simulink model "sampleModel7288_pp_1_1"  (R2018a)
settings: Solver=VariableStepAuto  StartTime=0.0  StopTime=10.0  RelTol=1e-3
undefined symbols (not defined in the file): DiscIntNeverNeededParam, sigbuilder_block
libraries: simulink x497
(part 5 of 10)

== system sampleModel7288_pp_1_1/cfblk302 ==
  cfblk1 : Inport
  Action Port : ActionPort  ActionType=then
  cfblk{4,7,9..10} (4 alike) : Delay
  cfblk3 : Delay  DelayLengthSource=Input port
      settings: InputPortMap=u0,p1
  cfblk5 : simulink/Discrete/Transfer Fcn Lead or Lag  PoleZ=0.95  ZeroZ=0.75  ICPrevOutput=0.0  ICPrevInput=0.0  DoSatur=off
      settings: SourceProductName=Simulink  SourceProductBaseCode=SL
  cfblk6 : simulink/Discrete/Difference  ICPrevInput=0.0  OutMin=[]  OutMax=[]  OutDataTypeStr=double  OutputDataTypeScalingMode=double  OutDataType=fixdt(1, 16)  OutScaling=2^-10  DoSatur=off
  cyemi_{1236..1243} (8 alike) : DataTypeConversion  OutDataTypeStr=double
  cfblk2 : Outport
  cfblk8 : Outport  Port=2
  wires:
  cfblk1/1 -> cfblk8/1
  cfblk7/1 -> cyemi_1236/1, cyemi_1237/1
  cfblk4/1 -> cyemi_1241/1, cyemi_1242/1
  cfblk6/1 -> cfblk2/1
  cyemi_1236/1 -> cfblk10/1
  cyemi_1237/1 -> cfblk3/1
  cyemi_1238/1 -> cfblk3/2
  cfblk9/1 -> cyemi_1238/1
  cyemi_1239/1 -> cfblk4/1
  cfblk10/1 -> cyemi_1239/1
  cyemi_1240/1 -> cfblk5/1
  cfblk3/1 -> cyemi_1240/1
  cyemi_1241/1 -> cfblk6/1
  cyemi_1242/1 -> cfblk7/1
  cyemi_1243/1 -> cfblk9/1
  cfblk5/1 -> cyemi_1243/1

== system sampleModel7288_pp_1_1/cfblk303 ==
  cfblk1 : Inport
  cfblk13 : Inport  Port=2
  cfblk14 : Inport  Port=3
  cfblk15 : Inport  Port=4
  Action Port : ActionPort  ActionType=else
  cfblk10 : Delay
  cfblk11 : DiscreteIntegrator  SampleTime=-1  OutDataTypeStr=double  ICPrevOutput=DiscIntNeverNeededParam  ICPrevScaledInput=DiscIntNeverNeededParam
  cfblk12 : simulink/Discrete/Transfer Fcn Lead or Lag  PoleZ=0.95  ZeroZ=0.75  ICPrevOutput=0.0  ICPrevInput=0.0  DoSatur=off
      settings: SourceProductName=Simulink  SourceProductBaseCode=SL
  cfblk17 : Delay
  cfblk3 : DiscreteFir
  cfblk4 : DiscreteFir
  cfblk5 : DiscreteStateSpace  SampleTime=-1
  cfblk6 : simulink/Discrete/Transfer Fcn Lead or Lag  PoleZ=0.95  ZeroZ=0.75  ICPrevOutput=0.0  ICPrevInput=0.0  DoSatur=off
      settings: SourceProductName=Simulink  SourceProductBaseCode=SL
  cfblk7 : Delay
  cfblk8 : DiscreteFilter
  cfblk9 : simulink/Discrete/Transfer Fcn Real Zero  ZeroZ=0.75  ICPrevInput=0.0  DoSatur=off
      settings: SourceProductName=Simulink  SourceProductBaseCode=SL
  cyemi_{1248..1258} (11 alike) : DataTypeConversion  OutDataTypeStr=double
  cfblk2 : Outport
  cfblk16 : Outport  Port=2
  wires:
  cfblk14/1 -> cfblk16/1
  cfblk3/1 -> cfblk2/1
  cyemi_1248/1 -> cfblk10/1
  cfblk8/1 -> cyemi_1248/1
  cyemi_1249/1 -> cfblk11/1
  cfblk9/1 -> cyemi_1249/1
  cyemi_1250/1 -> cfblk12/1
  cfblk5/1 -> cyemi_1250/1
  cyemi_1251/1 -> cfblk17/1
  cfblk11/1 -> cyemi_1251/1
  cyemi_1252/1 -> cfblk3/1
  cfblk7/1 -> cyemi_1252/1
  cyemi_1253/1 -> cfblk4/1
  cfblk12/1 -> cyemi_1253/1
  cyemi_1254/1 -> cfblk5/1
  cfblk1/1 -> cyemi_1254/1
  cyemi_1255/1 -> cfblk6/1
  cfblk4/1 -> cyemi_1255/1
  cyemi_1256/1 -> cfblk7/1
  cfblk6/1 -> cyemi_1256/1
  cyemi_1257/1 -> cfblk8/1
  cfblk15/1 -> cyemi_1257/1
  cyemi_1258/1 -> cfblk9/1
  cfblk17/1 -> cyemi_1258/1

== system sampleModel7288_pp_1_1/cfblk304 ==
  cfblk1 : Inport
  cfblk8 : Inport  Port=2
  Action Port : ActionPort  ActionType=then
  cfblk3 : simulink/Discrete/Transfer Fcn First Order  PoleZ=0.95  ICPrevOutput=0.0  DoSatur=off
      settings: SourceProductName=Simulink
  cfblk4 : simulink/Continuous/PID Controller (2DOF)  Controller=PID  TimeDomain=Discrete-time  SampleTime=-1  IntegratorMethod=Forward Euler  FilterMethod=Forward Euler  Form=Parallel  UseFilter=on  ControllerParametersSource=internal  P=1  I=1  D=0  N=100  b=1  c=1  InitialConditionSource=internal  InitialConditionForIntegrator=0  InitialConditionForFilter=0  ExternalReset=none  LimitOutput=off  UpperSaturationLimit=inf  LowerSaturationLimit=-inf  LinearizeAsGain=off  AntiWindupMode=none  Kb=1  TrackingMode=off  Kt=1  PParamMin=[]  PParamMax=[]  IParamMin=[]  IParamMax=[]  DParamMin=[]  DParamMax=[]  NParamMin=[]  NParamMax=[]  bParamMin=[]  bParamMax=[]  cParamMin=[]  cParamMax=[]  KbParamMin=[]  KbParamMax=[]  KtParamMin=[]  KtParamMax=[]  POutMin=[]  POutMax=[]  IOutMin=[]  IOutMax=[]  DOutMin=[]  DOutMax=[]  NOutMin=[]  NOutMax=[]  bOutMin=[]  bOutMax=[]  cOutMin=[]  cOutMax=[]  KbOutMin=[]  KbOutMax=[]  KtOutMin=[]  KtOutMax=[]  IntegratorOutMin=[]  IntegratorOutMax=[]  FilterOutMin=[]  FilterOutMax=[]  SumOutMin=[]  SumOutMax=[]  Sum1OutMin=[]  Sum1OutMax=[]  Sum2OutMin=[]  Sum2OutMax=[]  Sum3OutMin=[]  Sum3OutMax=[]  SumI1OutMin=[]  SumI1OutMax=[]  SumI2OutMin=[]  SumI2OutMax=[]  SumI3OutMin=[]  SumI3OutMax=[]  SumDOutMin=[]  SumDOutMax=[]  SaturationOutMin=[]  SaturationOutMax=[]  IntegratorContinuousStateAttributes=''  IntegratorStateMustResolveToSignalObject=off  IntegratorRTWStateStorageClass=Auto  FilterContinuousStateAttributes=''  FilterStateMustResolveToSignalObject=off  FilterRTWStateStorageClass=Auto  DifferentiatorICPrevScaledInput=0  DifferentiatorOutMin=[]  DifferentiatorOutMax=[]  FilterDiffOutCoefMin=[]  FilterDiffOutCoefMax=[]  SumDenOutMin=[]  SumDenOutMax=[]  SumNumOutMin=[]  SumNumOutMax=[]  ReciprocalOutMin=[]  ReciprocalOutMax=[]  DivideOutMin=[]  DivideOutMax=[]  TunerSelectOption=Transfer Function Based (PID Tuner App)
  cfblk5 : Delay  ShowEnablePort=on
      settings: InputPortMap=u0,e6
  cfblk6 : simulink/Discrete/Difference  ICPrevInput=0.0  OutMin=[]  OutMax=[]  OutDataTypeStr=double  OutputDataTypeScalingMode=double  OutDataType=fixdt(1, 16)  OutScaling=2^-10  DoSatur=off
  cfblk7 : DiscreteStateSpace  SampleTime=-1
  cfblk9 : Delay
  cyemi_{1261..1268} (8 alike) : DataTypeConversion  OutDataTypeStr=double
  cfblk2 : Outport
  wires:
  cfblk4/1 -> cfblk2/1
  cfblk8/1 -> cyemi_1261/1, cyemi_1262/1
  cyemi_1261/1 -> cfblk3/1
  cyemi_1262/1 -> cfblk4/1
  cyemi_1263/1 -> cfblk4/2
  cfblk6/1 -> cyemi_1263/1
  cyemi_1264/1 -> cfblk5/1
  cfblk1/1 -> cyemi_1264/1
  cyemi_1265/1 -> cfblk5/2
  cfblk9/1 -> cyemi_1265/1
  cyemi_1266/1 -> cfblk6/1
  cfblk3/1 -> cyemi_1266/1
  cyemi_1267/1 -> cfblk7/1
  cfblk5/1 -> cyemi_1267/1
  cyemi_1268/1 -> cfblk9/1
  cfblk7/1 -> cyemi_1268/1

== system sampleModel7288_pp_1_1/cfblk305 ==
  cfblk1 : Inport
  cfblk9 : Inport  Port=2
  cfblk10 : Inport  Port=3
  Action Port : ActionPort  ActionType=else
  cfblk13 : Subsystem  TreatAsAtomicUnit=on
  cfblk14 : Subsystem  TreatAsAtomicUnit=on
  cfblk15 : Delay
  cfblk16 : Delay
  cfblk3 : simulink/Discrete/Difference  ICPrevInput=0.0  OutMin=[]  OutMax=[]  OutDataTypeStr=double  OutputDataTypeScalingMode=double  OutDataType=fixdt(1, 16)  OutScaling=2^-10  DoSatur=off
  cfblk4 : simulink/Discrete/Transfer Fcn Lead or Lag  PoleZ=0.95  ZeroZ=0.75  ICPrevOutput=0.0  ICPrevInput=0.0  DoSatur=off
      settings: SourceProductName=Simulink  SourceProductBaseCode=SL
  cfblk5 : simulink/Discrete/Transfer Fcn First Order  PoleZ=0.95  ICPrevOutput=0.0  DoSatur=off
      settings: SourceProductName=Simulink
  cfblk6 : DiscreteFir
  cfblk7 : Delay  DelayLengthSource=Input port
      settings: InputPortMap=u0,p1
  cfblk8 : If  SampleTime=1
  cyemi_{1272..1273,1278..1280,1284..1292} (14 alike) : DataTypeConversion  OutDataTypeStr=double
  cfblk2 : Outport
  cfblk11 : Outport  Port=2
  cfblk12 : Outport  Port=3
  wires:
  cfblk13/1(cfblk2) -> cfblk11/1
  cfblk9/1 -> cfblk12/1
  cfblk10/1 -> cyemi_1272/1, cyemi_1278/1, cyemi_1279/1
  cfblk3/1 -> cyemi_1280/1, cyemi_1290/1
  cfblk13/2(cfblk7) -> cfblk2/1
  cfblk8/1 -> cfblk13/Action
  cfblk8/2 -> cfblk14/Action
  cyemi_1272/1 -> cfblk13/1(cfblk1)
  cyemi_1273/1 -> cfblk13/2(cfblk6)
  cfblk4/1 -> cyemi_1273/1
  cyemi_1278/1 -> cfblk14/1(cfblk1)
  cyemi_1279/1 -> cfblk14/2(cfblk5)
  cyemi_1280/1 -> cfblk14/3(cfblk6)
  cyemi_1284/1 -> cfblk15/1
  cfblk5/1 -> cyemi_1284/1
  cyemi_1285/1 -> cfblk16/1
  cfblk6/1 -> cyemi_1285/1
  cyemi_1286/1 -> cfblk3/1
  cfblk15/1 -> cyemi_1286/1
  cyemi_1287/1 -> cfblk4/1
  cfblk1/1 -> cyemi_1287/1
  cyemi_1288/1 -> cfblk5/1
  cfblk7/1 -> cyemi_1288/1
  cyemi_1289/1 -> cfblk6/1
  cfblk14/1(cfblk2) -> cyemi_1289/1
  cyemi_1290/1 -> cfblk7/1
  cyemi_1291/1 -> cfblk7/2
  cfblk14/2(cfblk7) -> cyemi_1291/1
  cyemi_1292/1 -> cfblk8/1
  cfblk16/1 -> cyemi_1292/1

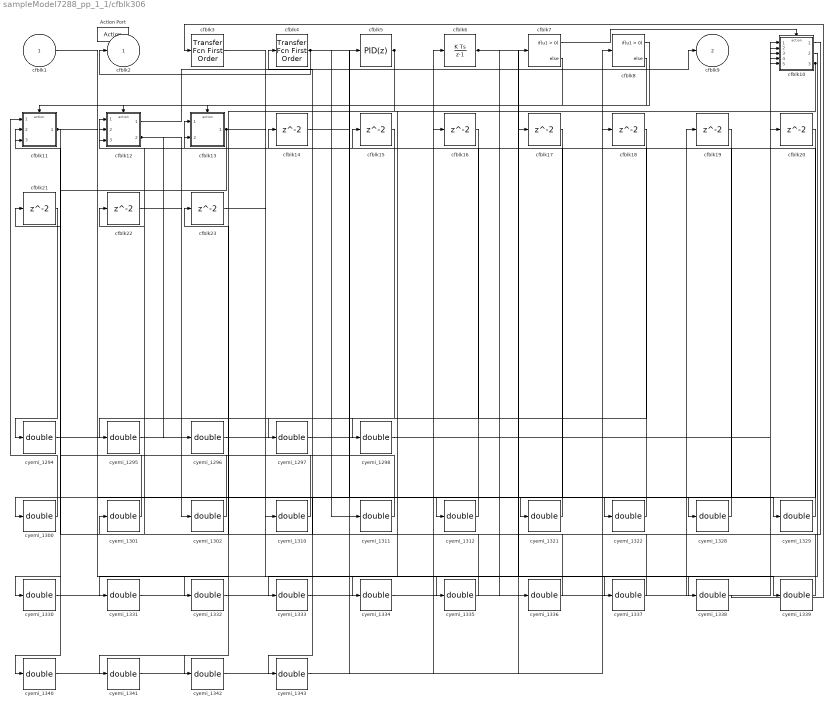
== system sampleModel7288_pp_1_1/cfblk306 ==
  cfblk1 : Inport
  Action Port : ActionPort  ActionType=then
  cfblk10 : Subsystem  TreatAsAtomicUnit=on
  cfblk11 : Subsystem  TreatAsAtomicUnit=on
  cfblk12 : Subsystem  TreatAsAtomicUnit=on
  cfblk13 : Subsystem  TreatAsAtomicUnit=on
  cfblk{14..23} (10 alike) : Delay
  cfblk3 : simulink/Discrete/Transfer Fcn First Order  PoleZ=0.95  ICPrevOutput=0.0  DoSatur=off
      settings: SourceProductName=Simulink
  cfblk4 : simulink/Discrete/Transfer Fcn First Order  PoleZ=0.95  ICPrevOutput=0.0  DoSatur=off
      settings: SourceProductName=Simulink
  cfblk5 : simulink/Continuous/PID Controller  Controller=PID  TimeDomain=Discrete-time  SampleTime=-1  IntegratorMethod=Forward Euler  FilterMethod=Forward Euler  Form=Parallel  UseFilter=on  ControllerParametersSource=internal  P=1  I=1  D=0  N=100  InitialConditionSource=internal  InitialConditionForIntegrator=0  InitialConditionForFilter=0  ExternalReset=none  LimitOutput=off  UpperSaturationLimit=inf  LowerSaturationLimit=-inf  LinearizeAsGain=off  AntiWindupMode=none  Kb=1  TrackingMode=off  Kt=1  PParamMin=[]  PParamMax=[]  IParamMin=[]  IParamMax=[]  DParamMin=[]  DParamMax=[]  NParamMin=[]  NParamMax=[]  KbParamMin=[]  KbParamMax=[]  KtParamMin=[]  KtParamMax=[]  POutMin=[]  POutMax=[]  IOutMin=[]  IOutMax=[]  DOutMin=[]  DOutMax=[]  NOutMin=[]  NOutMax=[]  KbOutMin=[]  KbOutMax=[]  KtOutMin=[]  KtOutMax=[]  IntegratorOutMin=[]  IntegratorOutMax=[]  FilterOutMin=[]  FilterOutMax=[]  SumOutMin=[]  SumOutMax=[]  SumI1OutMin=[]  SumI1OutMax=[]  SumI2OutMin=[]  SumI2OutMax=[]  SumI3OutMin=[]  SumI3OutMax=[]  SumDOutMin=[]  SumDOutMax=[]  SaturationOutMin=[]  SaturationOutMax=[]  IntegratorContinuousStateAttributes=''  IntegratorStateMustResolveToSignalObject=off  IntegratorRTWStateStorageClass=Auto  FilterContinuousStateAttributes=''  FilterStateMustResolveToSignalObject=off  FilterRTWStateStorageClass=Auto  DifferentiatorICPrevScaledInput=0  DifferentiatorOutMin=[]  DifferentiatorOutMax=[]  FilterDiffOutCoefMin=[]  FilterDiffOutCoefMax=[]  SumDenOutMin=[]  SumDenOutMax=[]  SumNumOutMin=[]  SumNumOutMax=[]  ReciprocalOutMin=[]  ReciprocalOutMax=[]  DivideOutMin=[]  DivideOutMax=[]  TunerSelectOption=Transfer Function Based (PID Tuner App)
  cfblk6 : DiscreteIntegrator  SampleTime=-1  OutDataTypeStr=double  ICPrevOutput=DiscIntNeverNeededParam  ICPrevScaledInput=DiscIntNeverNeededParam
  cfblk7 : If  SampleTime=1
  cfblk8 : If  SampleTime=1
  cyemi_{1294..1298,1300..1302,1310..1312,1321..1322,1328..1343} (29 alike) : DataTypeConversion  OutDataTypeStr=double
  cfblk2 : Outport
  cfblk9 : Outport  Port=2
  wires:
  cfblk5/1 -> cyemi_1331/1, cyemi_1332/1
  cfblk6/1 -> cyemi_1336/1, cyemi_1337/1, cyemi_1338/1
  cfblk4/1 -> cfblk2/1, cyemi_1311/1, cyemi_1312/1
  cfblk10/3(cfblk9) -> cyemi_1334/1, cyemi_1341/1
  cfblk11/1(cfblk2) -> cyemi_1328/1, cyemi_1340/1
  cfblk12/1(cfblk2) -> cfblk9/1
  cfblk13/1(cfblk2) -> cyemi_1329/1, cyemi_1330/1
  cfblk12/2(cfblk12) -> cyemi_1296/1, cyemi_1322/1
  cfblk7/1 -> cfblk10/Action
  cfblk7/2 -> cfblk11/Action
  cfblk8/1 -> cfblk12/Action
  cfblk8/2 -> cfblk13/Action
  cyemi_1294/1 -> cfblk10/1(cfblk1)
  cfblk21/1 -> cyemi_1294/1
  cyemi_1295/1 -> cfblk10/2(cfblk4)
  cfblk15/1 -> cyemi_1295/1
  cyemi_1296/1 -> cfblk10/3(cfblk5)
  cyemi_1297/1 -> cfblk10/4(cfblk6)
  cfblk18/1 -> cyemi_1297/1
  cyemi_1298/1 -> cfblk10/5(cfblk7)
  cfblk16/1 -> cyemi_1298/1
  cyemi_1300/1 -> cfblk11/1(cfblk1)
  cfblk17/1 -> cyemi_1300/1
  cyemi_1301/1 -> cfblk11/2(cfblk8)
  cfblk10/1(cfblk2) -> cyemi_1301/1
  cyemi_1302/1 -> cfblk11/3(cfblk9)
  cfblk22/1 -> cyemi_1302/1
  cyemi_1310/1 -> cfblk12/1(cfblk1)
  cfblk23/1 -> cyemi_1310/1
  cyemi_1311/1 -> cfblk12/2(cfblk10)
  cyemi_1312/1 -> cfblk12/3(cfblk11)
  cyemi_1321/1 -> cfblk13/1(cfblk1)
  cfblk14/1 -> cyemi_1321/1
  cyemi_1322/1 -> cfblk13/2(cfblk8)
  cyemi_1328/1 -> cfblk14/1
  cyemi_1329/1 -> cfblk15/1
  cyemi_1330/1 -> cfblk16/1
  cyemi_1331/1 -> cfblk17/1
  cyemi_1332/1 -> cfblk18/1
  cyemi_1333/1 -> cfblk19/1
  cfblk10/2(cfblk8) -> cyemi_1333/1
  cyemi_1334/1 -> cfblk20/1
  cyemi_1335/1 -> cfblk21/1
  cfblk3/1 -> cyemi_1335/1
  cyemi_1336/1 -> cfblk22/1
  cyemi_1337/1 -> cfblk23/1
  cyemi_1338/1 -> cfblk3/1
  cyemi_1339/1 -> cfblk4/1
  cfblk1/1 -> cyemi_1339/1
  cyemi_1340/1 -> cfblk5/1
  cyemi_1341/1 -> cfblk6/1
  cyemi_1342/1 -> cfblk7/1
  cfblk19/1 -> cyemi_1342/1
  cyemi_1343/1 -> cfblk8/1
  cfblk20/1 -> cyemi_1343/1

== system sampleModel7288_pp_1_1/cfblk307 ==
  cfblk1 : Inport
  cfblk12 : Inport  Port=2
  Action Port : ActionPort  ActionType=else
  cfblk10 : Delay  ShowEnablePort=on
      settings: InputPortMap=u0,e6
  cfblk11 : DiscreteFilter
  cfblk14 : Delay
  cfblk15 : Delay
  cfblk3 : Delay  DelayLengthSource=Input port
      settings: InputPortMap=u0,p1
  cfblk4 : DiscreteFilter
  cfblk5 : simulink/Continuous/PID Controller  Controller=PID  TimeDomain=Discrete-time  SampleTime=-1  IntegratorMethod=Forward Euler  FilterMethod=Forward Euler  Form=Parallel  UseFilter=on  ControllerParametersSource=internal  P=1  I=1  D=0  N=100  InitialConditionSource=internal  InitialConditionForIntegrator=0  InitialConditionForFilter=0  ExternalReset=none  LimitOutput=off  UpperSaturationLimit=inf  LowerSaturationLimit=-inf  LinearizeAsGain=off  AntiWindupMode=none  Kb=1  TrackingMode=off  Kt=1  PParamMin=[]  PParamMax=[]  IParamMin=[]  IParamMax=[]  DParamMin=[]  DParamMax=[]  NParamMin=[]  NParamMax=[]  KbParamMin=[]  KbParamMax=[]  KtParamMin=[]  KtParamMax=[]  POutMin=[]  POutMax=[]  IOutMin=[]  IOutMax=[]  DOutMin=[]  DOutMax=[]  NOutMin=[]  NOutMax=[]  KbOutMin=[]  KbOutMax=[]  KtOutMin=[]  KtOutMax=[]  IntegratorOutMin=[]  IntegratorOutMax=[]  FilterOutMin=[]  FilterOutMax=[]  SumOutMin=[]  SumOutMax=[]  SumI1OutMin=[]  SumI1OutMax=[]  SumI2OutMin=[]  SumI2OutMax=[]  SumI3OutMin=[]  SumI3OutMax=[]  SumDOutMin=[]  SumDOutMax=[]  SaturationOutMin=[]  SaturationOutMax=[]  IntegratorContinuousStateAttributes=''  IntegratorStateMustResolveToSignalObject=off  IntegratorRTWStateStorageClass=Auto  FilterContinuousStateAttributes=''  FilterStateMustResolveToSignalObject=off  FilterRTWStateStorageClass=Auto  DifferentiatorICPrevScaledInput=0  DifferentiatorOutMin=[]  DifferentiatorOutMax=[]  FilterDiffOutCoefMin=[]  FilterDiffOutCoefMax=[]  SumDenOutMin=[]  SumDenOutMax=[]  SumNumOutMin=[]  SumNumOutMax=[]  ReciprocalOutMin=[]  ReciprocalOutMax=[]  DivideOutMin=[]  DivideOutMax=[]  TunerSelectOption=Transfer Function Based (PID Tuner App)
  cfblk6 : DiscreteStateSpace  SampleTime=-1
  cfblk7 : UnitDelay  SampleTime=-1
  cfblk8 : Delay
  cfblk9 : DiscreteIntegrator  SampleTime=-1  OutDataTypeStr=double  ICPrevOutput=DiscIntNeverNeededParam  ICPrevScaledInput=DiscIntNeverNeededParam
  cyemi_{1346..1358} (13 alike) : DataTypeConversion  OutDataTypeStr=double
  cfblk2 : Outport
  cfblk13 : Outport  Port=2
  wires:
  cfblk1/1 -> cyemi_1352/1, cyemi_1358/1
  cfblk7/1 -> cfblk13/1
  cfblk5/1 -> cfblk2/1, cyemi_1355/1
  cyemi_1346/1 -> cfblk10/1
  cfblk14/1 -> cyemi_1346/1
  cyemi_1347/1 -> cfblk10/2
  cfblk3/1 -> cyemi_1347/1
  cyemi_1348/1 -> cfblk11/1
  cfblk9/1 -> cyemi_1348/1
  cyemi_1349/1 -> cfblk14/1
  cfblk8/1 -> cyemi_1349/1
  cyemi_1350/1 -> cfblk15/1
  cfblk6/1 -> cyemi_1350/1
  cyemi_1351/1 -> cfblk3/1
  cfblk12/1 -> cyemi_1351/1
  cyemi_1352/1 -> cfblk3/2
  cyemi_1353/1 -> cfblk4/1
  cfblk11/1 -> cyemi_1353/1
  cyemi_1354/1 -> cfblk5/1
  cfblk15/1 -> cyemi_1354/1
  cyemi_1355/1 -> cfblk6/1
  cyemi_1356/1 -> cfblk7/1
  cfblk4/1 -> cyemi_1356/1
  cyemi_1357/1 -> cfblk8/1
  cfblk10/1 -> cyemi_1357/1
  cyemi_1358/1 -> cfblk9/1

== system sampleModel7288_pp_1_1/cfblk308 ==
  cfblk1 : Inport
  Action Port : ActionPort  ActionType=then
  cfblk3 : DiscreteStateSpace  SampleTime=-1
  cfblk4 : DiscreteStateSpace  SampleTime=-1
  cfblk5 : DiscreteFilter
  cfblk6 : simulink/Discrete/Tapped Delay  vinit=0.0  samptime=-1  NumDelays=1  DelayOrder=Oldest  includeCurrent=off
  cfblk7 : DiscreteIntegrator  SampleTime=-1  OutDataTypeStr=double  ICPrevOutput=DiscIntNeverNeededParam  ICPrevScaledInput=DiscIntNeverNeededParam
  cfblk8 : Delay  ShowEnablePort=on
      settings: InputPortMap=u0,e6
  cfblk9 : simulink/Discrete/Transfer Fcn Lead or Lag  PoleZ=0.95  ZeroZ=0.75  ICPrevOutput=0.0  ICPrevInput=0.0  DoSatur=off
      settings: SourceProductName=Simulink  SourceProductBaseCode=SL
  cyemi_{1360..1367} (8 alike) : DataTypeConversion  OutDataTypeStr=double
  cfblk2 : Outport
  cfblk10 : Outport  Port=2
  wires:
  cfblk3/1 -> cyemi_1366/1, cyemi_1367/1
  cfblk7/1 -> cyemi_1362/1, cyemi_1363/1
  cfblk4/1 -> cfblk10/1
  cfblk8/1 -> cfblk2/1
  cyemi_1360/1 -> cfblk3/1
  cfblk5/1 -> cyemi_1360/1
  cyemi_1361/1 -> cfblk4/1
  cfblk9/1 -> cyemi_1361/1
  cyemi_1362/1 -> cfblk5/1
  cyemi_1363/1 -> cfblk6/1
  cyemi_1364/1 -> cfblk7/1
  cfblk1/1 -> cyemi_1364/1
  cyemi_1365/1 -> cfblk8/1
  cfblk6/1 -> cyemi_1365/1
  cyemi_1366/1 -> cfblk8/2
  cyemi_1367/1 -> cfblk9/1

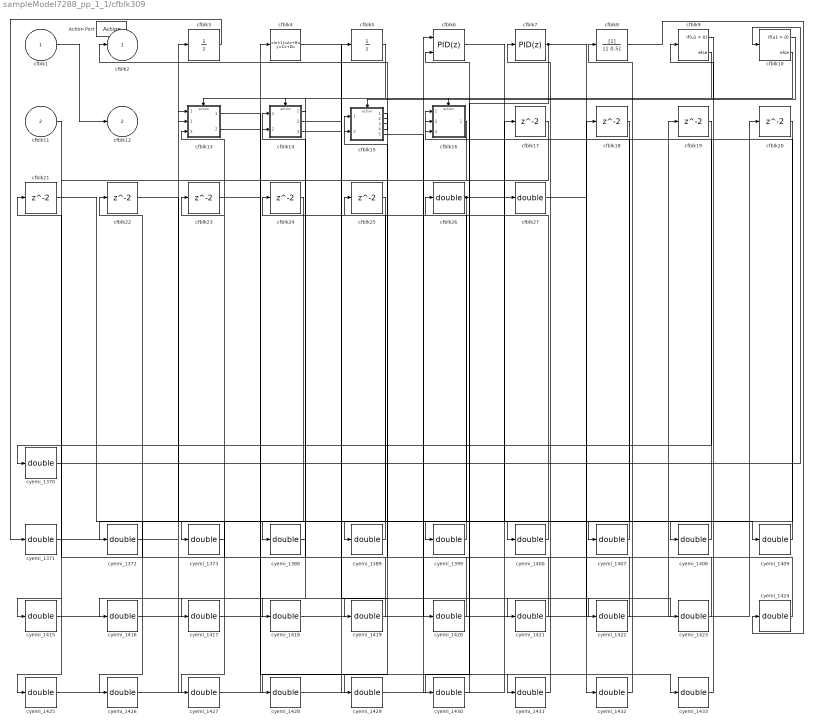
== system sampleModel7288_pp_1_1/cfblk309 ==
  cfblk1 : Inport
  cfblk11 : Inport  Port=2
  Action Port : ActionPort  ActionType=else
  cfblk10 : If  SampleTime=1
  cfblk13 : Subsystem  TreatAsAtomicUnit=on
  cfblk14 : Subsystem  TreatAsAtomicUnit=on
  cfblk15 : Subsystem  TreatAsAtomicUnit=on
  cfblk16 : Subsystem  TreatAsAtomicUnit=on
  cfblk{17..25} (9 alike) : Delay
  cfblk26 : DataTypeConversion  OutDataTypeStr=double
  cfblk27 : DataTypeConversion  OutDataTypeStr=double
  cfblk3 : UnitDelay  SampleTime=-1
  cfblk4 : DiscreteStateSpace  SampleTime=-1
  cfblk5 : UnitDelay  SampleTime=-1
  cfblk6 : simulink/Continuous/PID Controller (2DOF)  Controller=PID  TimeDomain=Discrete-time  SampleTime=-1  IntegratorMethod=Forward Euler  FilterMethod=Forward Euler  Form=Parallel  UseFilter=on  ControllerParametersSource=internal  P=1  I=1  D=0  N=100  b=1  c=1  InitialConditionSource=internal  InitialConditionForIntegrator=0  InitialConditionForFilter=0  ExternalReset=none  LimitOutput=off  UpperSaturationLimit=inf  LowerSaturationLimit=-inf  LinearizeAsGain=off  AntiWindupMode=none  Kb=1  TrackingMode=off  Kt=1  PParamMin=[]  PParamMax=[]  IParamMin=[]  IParamMax=[]  DParamMin=[]  DParamMax=[]  NParamMin=[]  NParamMax=[]  bParamMin=[]  bParamMax=[]  cParamMin=[]  cParamMax=[]  KbParamMin=[]  KbParamMax=[]  KtParamMin=[]  KtParamMax=[]  POutMin=[]  POutMax=[]  IOutMin=[]  IOutMax=[]  DOutMin=[]  DOutMax=[]  NOutMin=[]  NOutMax=[]  bOutMin=[]  bOutMax=[]  cOutMin=[]  cOutMax=[]  KbOutMin=[]  KbOutMax=[]  KtOutMin=[]  KtOutMax=[]  IntegratorOutMin=[]  IntegratorOutMax=[]  FilterOutMin=[]  FilterOutMax=[]  SumOutMin=[]  SumOutMax=[]  Sum1OutMin=[]  Sum1OutMax=[]  Sum2OutMin=[]  Sum2OutMax=[]  Sum3OutMin=[]  Sum3OutMax=[]  SumI1OutMin=[]  SumI1OutMax=[]  SumI2OutMin=[]  SumI2OutMax=[]  SumI3OutMin=[]  SumI3OutMax=[]  SumDOutMin=[]  SumDOutMax=[]  SaturationOutMin=[]  SaturationOutMax=[]  IntegratorContinuousStateAttributes=''  IntegratorStateMustResolveToSignalObject=off  IntegratorRTWStateStorageClass=Auto  FilterContinuousStateAttributes=''  FilterStateMustResolveToSignalObject=off  FilterRTWStateStorageClass=Auto  DifferentiatorICPrevScaledInput=0  DifferentiatorOutMin=[]  DifferentiatorOutMax=[]  FilterDiffOutCoefMin=[]  FilterDiffOutCoefMax=[]  SumDenOutMin=[]  SumDenOutMax=[]  SumNumOutMin=[]  SumNumOutMax=[]  ReciprocalOutMin=[]  ReciprocalOutMax=[]  DivideOutMin=[]  DivideOutMax=[]  TunerSelectOption=Transfer Function Based (PID Tuner App)
  cfblk7 : simulink/Continuous/PID Controller  Controller=PID  TimeDomain=Discrete-time  SampleTime=-1  IntegratorMethod=Forward Euler  FilterMethod=Forward Euler  Form=Parallel  UseFilter=on  ControllerParametersSource=internal  P=1  I=1  D=0  N=100  InitialConditionSource=internal  InitialConditionForIntegrator=0  InitialConditionForFilter=0  ExternalReset=none  LimitOutput=off  UpperSaturationLimit=inf  LowerSaturationLimit=-inf  LinearizeAsGain=off  AntiWindupMode=none  Kb=1  TrackingMode=off  Kt=1  PParamMin=[]  PParamMax=[]  IParamMin=[]  IParamMax=[]  DParamMin=[]  DParamMax=[]  NParamMin=[]  NParamMax=[]  KbParamMin=[]  KbParamMax=[]  KtParamMin=[]  KtParamMax=[]  POutMin=[]  POutMax=[]  IOutMin=[]  IOutMax=[]  DOutMin=[]  DOutMax=[]  NOutMin=[]  NOutMax=[]  KbOutMin=[]  KbOutMax=[]  KtOutMin=[]  KtOutMax=[]  IntegratorOutMin=[]  IntegratorOutMax=[]  FilterOutMin=[]  FilterOutMax=[]  SumOutMin=[]  SumOutMax=[]  SumI1OutMin=[]  SumI1OutMax=[]  SumI2OutMin=[]  SumI2OutMax=[]  SumI3OutMin=[]  SumI3OutMax=[]  SumDOutMin=[]  SumDOutMax=[]  SaturationOutMin=[]  SaturationOutMax=[]  IntegratorContinuousStateAttributes=''  IntegratorStateMustResolveToSignalObject=off  IntegratorRTWStateStorageClass=Auto  FilterContinuousStateAttributes=''  FilterStateMustResolveToSignalObject=off  FilterRTWStateStorageClass=Auto  DifferentiatorICPrevScaledInput=0  DifferentiatorOutMin=[]  DifferentiatorOutMax=[]  FilterDiffOutCoefMin=[]  FilterDiffOutCoefMax=[]  SumDenOutMin=[]  SumDenOutMax=[]  SumNumOutMin=[]  SumNumOutMax=[]  ReciprocalOutMin=[]  ReciprocalOutMax=[]  DivideOutMin=[]  DivideOutMax=[]  TunerSelectOption=Transfer Function Based (PID Tuner App)
  cfblk8 : DiscreteFilter
  cfblk9 : If  SampleTime=1
  cyemi_{1370..1373,1388..1389,1399..1400,1407..1409,1415..1433} (30 alike) : DataTypeConversion  OutDataTypeStr=double
  cfblk2 : Outport
  cfblk12 : Outport  Port=2
  wires:
  cfblk1/1 -> cfblk12/1
  cfblk7/1 -> cyemi_1423/1, cyemi_1430/1
  cfblk15/4(cfblk10) -> cfblk2/1
  cfblk9/1 -> cfblk13/Action
  cfblk9/2 -> cfblk14/Action
  cfblk10/1 -> cfblk15/Action
  cfblk10/2 -> cfblk16/Action
  cfblk26/1 -> cyemi_1409/1, cyemi_1427/1
  cyemi_1370/1 -> cfblk10/1
  cfblk19/1 -> cyemi_1370/1
  cyemi_1371/1 -> cfblk13/1(cfblk1)
  cfblk3/1 -> cyemi_1371/1
  cyemi_1372/1 -> cfblk13/2(cfblk15)
  cfblk25/1 -> cyemi_1372/1
  cyemi_1373/1 -> cfblk13/3(cfblk16)
  cfblk20/1 -> cyemi_1373/1
  cyemi_1388/1 -> cfblk14/1(cfblk1)
  cfblk17/1 -> cyemi_1388/1
  cyemi_1389/1 -> cfblk14/2(cfblk12)
  cfblk21/1 -> cyemi_1389/1
  cyemi_1399/1 -> cfblk15/1(cfblk1)
  cfblk18/1 -> cyemi_1399/1
  cyemi_1400/1 -> cfblk15/2(cfblk7)
  cfblk4/1 -> cyemi_1400/1
  cyemi_1407/1 -> cfblk16/1(cfblk1)
  cfblk6/1 -> cyemi_1407/1
  cyemi_1408/1 -> cfblk16/2(cfblk7)
  cfblk22/1 -> cyemi_1408/1
  cyemi_1409/1 -> cfblk16/3(cfblk8)
  cyemi_1415/1 -> cfblk17/1
  cfblk16/1(cfblk2) -> cyemi_1415/1
  cyemi_1416/1 -> cfblk18/1
  cfblk14/1(cfblk2) -> cyemi_1416/1
  cyemi_1417/1 -> cfblk19/1
  cfblk15/1(cfblk2) -> cyemi_1417/1
  cyemi_1418/1 -> cfblk20/1
  cfblk5/1 -> cyemi_1418/1
  cyemi_1419/1 -> cfblk21/1
  cfblk15/3(cfblk9) -> cyemi_1419/1
  cyemi_1420/1 -> cfblk22/1
  cfblk15/5(cfblk11) -> cyemi_1420/1
  cyemi_1421/1 -> cfblk23/1
  cfblk14/2(cfblk13) -> cyemi_1421/1
  cyemi_1422/1 -> cfblk24/1
  cfblk14/3(cfblk14) -> cyemi_1422/1
  cyemi_1423/1 -> cfblk25/1
  cyemi_1424/1 -> cfblk26/1
  cfblk8/1 -> cyemi_1424/1
  cyemi_1425/1 -> cfblk27/1
  cfblk11/1 -> cyemi_1425/1
  cyemi_1426/1 -> cfblk3/1
  cfblk24/1 -> cyemi_1426/1
  cyemi_1427/1 -> cfblk4/1
  cyemi_1428/1 -> cfblk5/1
  cfblk15/2(cfblk8) -> cyemi_1428/1
  cyemi_1429/1 -> cfblk6/1
  cfblk13/1(cfblk2) -> cyemi_1429/1
  cyemi_1430/1 -> cfblk6/2
  cyemi_1431/1 -> cfblk7/1
  cfblk13/2(cfblk17) -> cyemi_1431/1
  cyemi_1432/1 -> cfblk8/1
  cfblk27/1 -> cyemi_1432/1
  cyemi_1433/1 -> cfblk9/1
  cfblk23/1 -> cyemi_1433/1

== system sampleModel7288_pp_1_1/cfblk310 ==
  cfblk1 : Inport
  cfblk14 : Inport  Port=2
  cfblk15 : Inport  Port=3
  Action Port : ActionPort  ActionType=then
  cfblk10 : UnitDelay  SampleTime=-1
  cfblk11 : DiscreteFir
  cfblk12 : UnitDelay  SampleTime=-1
  cfblk13 : If  SampleTime=1
  cfblk16 : Subsystem  TreatAsAtomicUnit=on
  cfblk17 : Subsystem  TreatAsAtomicUnit=on
  cfblk18 : Delay
  cfblk19 : Delay
  cfblk3 : simulink/Discrete/Tapped Delay  vinit=0.0  samptime=-1  NumDelays=1  DelayOrder=Oldest  includeCurrent=off
  cfblk4 : simulink/Continuous/PID Controller (2DOF)  Controller=PID  TimeDomain=Discrete-time  SampleTime=-1  IntegratorMethod=Forward Euler  FilterMethod=Forward Euler  Form=Parallel  UseFilter=on  ControllerParametersSource=internal  P=1  I=1  D=0  N=100  b=1  c=1  InitialConditionSource=internal  InitialConditionForIntegrator=0  InitialConditionForFilter=0  ExternalReset=none  LimitOutput=off  UpperSaturationLimit=inf  LowerSaturationLimit=-inf  LinearizeAsGain=off  AntiWindupMode=none  Kb=1  TrackingMode=off  Kt=1  PParamMin=[]  PParamMax=[]  IParamMin=[]  IParamMax=[]  DParamMin=[]  DParamMax=[]  NParamMin=[]  NParamMax=[]  bParamMin=[]  bParamMax=[]  cParamMin=[]  cParamMax=[]  KbParamMin=[]  KbParamMax=[]  KtParamMin=[]  KtParamMax=[]  POutMin=[]  POutMax=[]  IOutMin=[]  IOutMax=[]  DOutMin=[]  DOutMax=[]  NOutMin=[]  NOutMax=[]  bOutMin=[]  bOutMax=[]  cOutMin=[]  cOutMax=[]  KbOutMin=[]  KbOutMax=[]  KtOutMin=[]  KtOutMax=[]  IntegratorOutMin=[]  IntegratorOutMax=[]  FilterOutMin=[]  FilterOutMax=[]  SumOutMin=[]  SumOutMax=[]  Sum1OutMin=[]  Sum1OutMax=[]  Sum2OutMin=[]  Sum2OutMax=[]  Sum3OutMin=[]  Sum3OutMax=[]  SumI1OutMin=[]  SumI1OutMax=[]  SumI2OutMin=[]  SumI2OutMax=[]  SumI3OutMin=[]  SumI3OutMax=[]  SumDOutMin=[]  SumDOutMax=[]  SaturationOutMin=[]  SaturationOutMax=[]  IntegratorContinuousStateAttributes=''  IntegratorStateMustResolveToSignalObject=off  IntegratorRTWStateStorageClass=Auto  FilterContinuousStateAttributes=''  FilterStateMustResolveToSignalObject=off  FilterRTWStateStorageClass=Auto  DifferentiatorICPrevScaledInput=0  DifferentiatorOutMin=[]  DifferentiatorOutMax=[]  FilterDiffOutCoefMin=[]  FilterDiffOutCoefMax=[]  SumDenOutMin=[]  SumDenOutMax=[]  SumNumOutMin=[]  SumNumOutMax=[]  ReciprocalOutMin=[]  ReciprocalOutMax=[]  DivideOutMin=[]  DivideOutMax=[]  TunerSelectOption=Transfer Function Based (PID Tuner App)
  cfblk5 : DiscreteStateSpace  SampleTime=-1
  cfblk6 : simulink/Discrete/Transfer Fcn Lead or Lag  PoleZ=0.95  ZeroZ=0.75  ICPrevOutput=0.0  ICPrevInput=0.0  DoSatur=off
      settings: SourceProductName=Simulink  SourceProductBaseCode=SL
  cfblk7 : UnitDelay  SampleTime=-1
  cfblk8 : simulink/Discrete/Tapped Delay  vinit=0.0  samptime=-1  NumDelays=1  DelayOrder=Oldest  includeCurrent=off
  cfblk9 : DiscreteZeroPole  Poles=[0 0.5]  Gain=1  SampleTime=-1
  cyemi_{1438..1442,1468..1469,1483..1492} (17 alike) : DataTypeConversion  OutDataTypeStr=double
  cfblk2 : Outport
  wires:
  cfblk11/1 -> cfblk2/1
  cfblk13/1 -> cfblk16/Action
  cfblk13/2 -> cfblk17/Action
  cyemi_1438/1 -> cfblk10/1
  cfblk19/1 -> cyemi_1438/1
  cyemi_1439/1 -> cfblk11/1
  cfblk3/1 -> cyemi_1439/1
  cyemi_1440/1 -> cfblk12/1
  cfblk8/1 -> cyemi_1440/1
  cyemi_1441/1 -> cfblk13/1
  cfblk14/1 -> cyemi_1441/1
  cyemi_1442/1 -> cfblk16/1(cfblk1)
  cfblk10/1 -> cyemi_1442/1
  cyemi_1468/1 -> cfblk17/1(cfblk1)
  cfblk18/1 -> cyemi_1468/1
  cyemi_1469/1 -> cfblk17/2(cfblk10)
  cfblk5/1 -> cyemi_1469/1
  cyemi_1483/1 -> cfblk18/1
  cfblk4/1 -> cyemi_1483/1
  cyemi_1484/1 -> cfblk19/1
  cfblk16/1(cfblk2) -> cyemi_1484/1
  cyemi_1485/1 -> cfblk3/1
  cfblk7/1 -> cyemi_1485/1
  cyemi_1486/1 -> cfblk4/1
  cfblk16/2(cfblk17) -> cyemi_1486/1
  cyemi_1487/1 -> cfblk4/2
  cfblk17/1(cfblk2) -> cyemi_1487/1
  cyemi_1488/1 -> cfblk5/1
  cfblk12/1 -> cyemi_1488/1
  cyemi_1489/1 -> cfblk6/1
  cfblk1/1 -> cyemi_1489/1
  cyemi_1490/1 -> cfblk7/1
  cfblk9/1 -> cyemi_1490/1
  cyemi_1491/1 -> cfblk8/1
  cfblk6/1 -> cyemi_1491/1
  cyemi_1492/1 -> cfblk9/1
  cfblk15/1 -> cyemi_1492/1

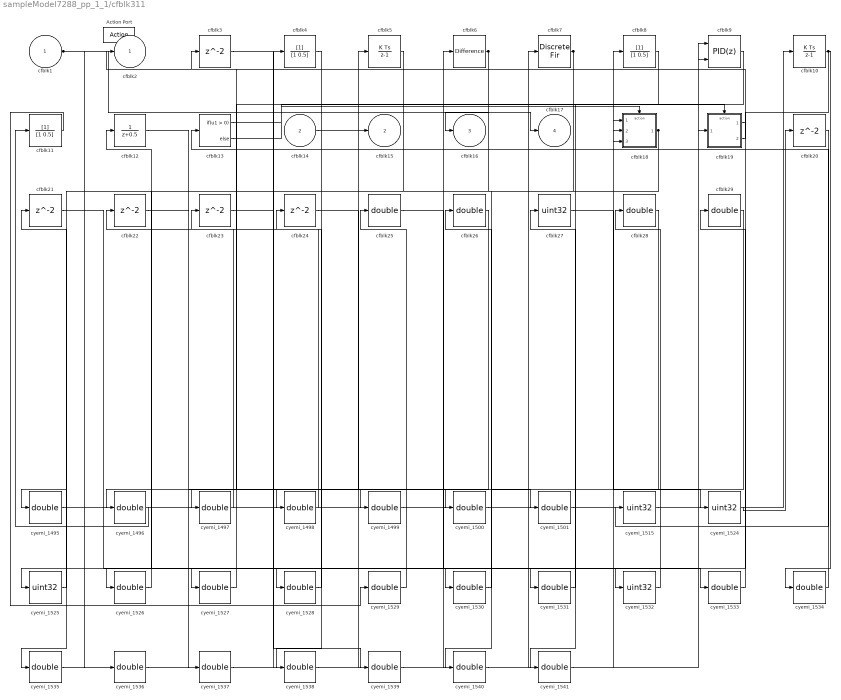
== system sampleModel7288_pp_1_1/cfblk311 ==
  cfblk1 : Inport
  cfblk14 : Inport  Port=2
  Action Port : ActionPort  ActionType=else
  cfblk10 : DiscreteIntegrator  SampleTime=-1  OutDataTypeStr=double  ICPrevOutput=DiscIntNeverNeededParam  ICPrevScaledInput=DiscIntNeverNeededParam
  cfblk11 : DiscreteFilter
  cfblk12 : DiscreteTransferFcn
  cfblk13 : If  SampleTime=1
  cfblk18 : Subsystem  TreatAsAtomicUnit=on
  cfblk19 : Subsystem  TreatAsAtomicUnit=on
  cfblk{3,20..24} (6 alike) : Delay
  cfblk{25..26,28..29} (4 alike) : DataTypeConversion  OutDataTypeStr=double
  cfblk27 : DataTypeConversion  OutDataTypeStr=uint32
  cfblk4 : DiscreteFilter
  cfblk5 : DiscreteIntegrator  SampleTime=-1  OutDataTypeStr=double  ICPrevOutput=DiscIntNeverNeededParam  ICPrevScaledInput=DiscIntNeverNeededParam
  cfblk6 : simulink/Discrete/Difference  ICPrevInput=0.0  OutMin=[]  OutMax=[]  OutDataTypeStr=double  OutputDataTypeScalingMode=double  OutDataType=fixdt(1, 16)  OutScaling=2^-10  DoSatur=off
  cfblk7 : DiscreteFir
  cfblk8 : DiscreteFilter
  cfblk9 : simulink/Continuous/PID Controller (2DOF)  Controller=PID  TimeDomain=Discrete-time  SampleTime=-1  IntegratorMethod=Forward Euler  FilterMethod=Forward Euler  Form=Parallel  UseFilter=on  ControllerParametersSource=internal  P=1  I=1  D=0  N=100  b=1  c=1  InitialConditionSource=internal  InitialConditionForIntegrator=0  InitialConditionForFilter=0  ExternalReset=none  LimitOutput=off  UpperSaturationLimit=inf  LowerSaturationLimit=-inf  LinearizeAsGain=off  AntiWindupMode=none  Kb=1  TrackingMode=off  Kt=1  PParamMin=[]  PParamMax=[]  IParamMin=[]  IParamMax=[]  DParamMin=[]  DParamMax=[]  NParamMin=[]  NParamMax=[]  bParamMin=[]  bParamMax=[]  cParamMin=[]  cParamMax=[]  KbParamMin=[]  KbParamMax=[]  KtParamMin=[]  KtParamMax=[]  POutMin=[]  POutMax=[]  IOutMin=[]  IOutMax=[]  DOutMin=[]  DOutMax=[]  NOutMin=[]  NOutMax=[]  bOutMin=[]  bOutMax=[]  cOutMin=[]  cOutMax=[]  KbOutMin=[]  KbOutMax=[]  KtOutMin=[]  KtOutMax=[]  IntegratorOutMin=[]  IntegratorOutMax=[]  FilterOutMin=[]  FilterOutMax=[]  SumOutMin=[]  SumOutMax=[]  Sum1OutMin=[]  Sum1OutMax=[]  Sum2OutMin=[]  Sum2OutMax=[]  Sum3OutMin=[]  Sum3OutMax=[]  SumI1OutMin=[]  SumI1OutMax=[]  SumI2OutMin=[]  SumI2OutMax=[]  SumI3OutMin=[]  SumI3OutMax=[]  SumDOutMin=[]  SumDOutMax=[]  SaturationOutMin=[]  SaturationOutMax=[]  IntegratorContinuousStateAttributes=''  IntegratorStateMustResolveToSignalObject=off  IntegratorRTWStateStorageClass=Auto  FilterContinuousStateAttributes=''  FilterStateMustResolveToSignalObject=off  FilterRTWStateStorageClass=Auto  DifferentiatorICPrevScaledInput=0  DifferentiatorOutMin=[]  DifferentiatorOutMax=[]  FilterDiffOutCoefMin=[]  FilterDiffOutCoefMax=[]  SumDenOutMin=[]  SumDenOutMax=[]  SumNumOutMin=[]  SumNumOutMax=[]  ReciprocalOutMin=[]  ReciprocalOutMax=[]  DivideOutMin=[]  DivideOutMax=[]  TunerSelectOption=Transfer Function Based (PID Tuner App)
  cyemi_{1495..1501,1526..1531,1533..1541} (22 alike) : DataTypeConversion  OutDataTypeStr=double
  cyemi_{1515,1524..1525,1532} (4 alike) : DataTypeConversion  OutDataTypeStr=uint32
  cfblk2 : Outport
  cfblk15 : Outport  Port=2
  cfblk16 : Outport  Port=3
  cfblk17 : Outport  Port=4
  wires:
  cfblk6/1 -> cfblk16/1, cyemi_1526/1
  cfblk18/1(cfblk2) -> cyemi_1530/1, cyemi_1538/1
  cfblk14/1 -> cfblk15/1
  cfblk7/1 -> cyemi_1495/1, cyemi_1528/1
  cfblk10/1 -> cyemi_1527/1, cyemi_1534/1
  cfblk1/1 -> cfblk17/1, cyemi_1536/1
  cfblk19/2(cfblk8) -> cfblk2/1
  cfblk13/1 -> cfblk18/Action
  cfblk13/2 -> cfblk19/Action
  cyemi_1495/1 -> cfblk10/1
  cyemi_1496/1 -> cfblk11/1
  cfblk26/1 -> cyemi_1496/1
  cyemi_1497/1 -> cfblk12/1
  cfblk8/1 -> cyemi_1497/1
  cyemi_1498/1 -> cfblk13/1
  cfblk4/1 -> cyemi_1498/1
  cyemi_1499/1 -> cfblk18/1(cfblk1)
  cfblk22/1 -> cyemi_1499/1
  cyemi_1500/1 -> cfblk18/2(cfblk13)
  cfblk23/1 -> cyemi_1500/1
  cyemi_1501/1 -> cfblk18/3(cfblk14)
  cfblk24/1 -> cyemi_1501/1
  cyemi_1515/1 -> cfblk19/1(cfblk1)
  cfblk20/1 -> cyemi_1515/1
  cyemi_1524/1 -> cfblk20/1
  cfblk27/1 -> cyemi_1524/1
  cyemi_1525/1 -> cfblk21/1
  cfblk19/1(cfblk2) -> cyemi_1525/1
  cyemi_1526/1 -> cfblk22/1
  cyemi_1527/1 -> cfblk23/1
  cyemi_1528/1 -> cfblk24/1
  cyemi_1529/1 -> cfblk25/1
  cfblk11/1 -> cyemi_1529/1
  cyemi_1530/1 -> cfblk26/1
  cyemi_1531/1 -> cfblk27/1
  cfblk9/1 -> cyemi_1531/1
  cyemi_1532/1 -> cfblk28/1
  cfblk21/1 -> cyemi_1532/1
  cyemi_1533/1 -> cfblk29/1
  cfblk25/1 -> cyemi_1533/1
  cyemi_1534/1 -> cfblk3/1
  cyemi_1535/1 -> cfblk4/1
  cfblk5/1 -> cyemi_1535/1
  cyemi_1536/1 -> cfblk5/1
  cyemi_1537/1 -> cfblk6/1
  cfblk12/1 -> cyemi_1537/1
  cyemi_1538/1 -> cfblk7/1
  cyemi_1539/1 -> cfblk8/1
  cfblk3/1 -> cyemi_1539/1
  cyemi_1540/1 -> cfblk9/1
  cfblk28/1 -> cyemi_1540/1
  cyemi_1541/1 -> cfblk9/2
  cfblk29/1 -> cyemi_1541/1

== system sampleModel7288_pp_1_1/cfblk312 ==
  cfblk1 : Inport
  Action Port : ActionPort  ActionType=then
  cfblk10 : UnitDelay  SampleTime=-1
  cfblk11 : DiscreteTransferFcn
  cfblk12 : If  SampleTime=1
  cfblk15 : Subsystem  TreatAsAtomicUnit=on
  cfblk16 : Subsystem  TreatAsAtomicUnit=on
  cfblk17 : Delay
  cfblk18 : Delay
  cfblk19 : Delay
  cfblk3 : DiscreteIntegrator  SampleTime=-1  OutDataTypeStr=double  ICPrevOutput=DiscIntNeverNeededParam  ICPrevScaledInput=DiscIntNeverNeededParam
  cfblk4 : DiscreteFir
  cfblk5 : simulink/Discrete/Tapped Delay  vinit=0.0  samptime=-1  NumDelays=1  DelayOrder=Oldest  includeCurrent=off
  cfblk6 : UnitDelay  SampleTime=-1
  cfblk7 : simulink/Continuous/PID Controller (2DOF)  Controller=PID  TimeDomain=Discrete-time  SampleTime=-1  IntegratorMethod=Forward Euler  FilterMethod=Forward Euler  Form=Parallel  UseFilter=on  ControllerParametersSource=internal  P=1  I=1  D=0  N=100  b=1  c=1  InitialConditionSource=internal  InitialConditionForIntegrator=0  InitialConditionForFilter=0  ExternalReset=none  LimitOutput=off  UpperSaturationLimit=inf  LowerSaturationLimit=-inf  LinearizeAsGain=off  AntiWindupMode=none  Kb=1  TrackingMode=off  Kt=1  PParamMin=[]  PParamMax=[]  IParamMin=[]  IParamMax=[]  DParamMin=[]  DParamMax=[]  NParamMin=[]  NParamMax=[]  bParamMin=[]  bParamMax=[]  cParamMin=[]  cParamMax=[]  KbParamMin=[]  KbParamMax=[]  KtParamMin=[]  KtParamMax=[]  POutMin=[]  POutMax=[]  IOutMin=[]  IOutMax=[]  DOutMin=[]  DOutMax=[]  NOutMin=[]  NOutMax=[]  bOutMin=[]  bOutMax=[]  cOutMin=[]  cOutMax=[]  KbOutMin=[]  KbOutMax=[]  KtOutMin=[]  KtOutMax=[]  IntegratorOutMin=[]  IntegratorOutMax=[]  FilterOutMin=[]  FilterOutMax=[]  SumOutMin=[]  SumOutMax=[]  Sum1OutMin=[]  Sum1OutMax=[]  Sum2OutMin=[]  Sum2OutMax=[]  Sum3OutMin=[]  Sum3OutMax=[]  SumI1OutMin=[]  SumI1OutMax=[]  SumI2OutMin=[]  SumI2OutMax=[]  SumI3OutMin=[]  SumI3OutMax=[]  SumDOutMin=[]  SumDOutMax=[]  SaturationOutMin=[]  SaturationOutMax=[]  IntegratorContinuousStateAttributes=''  IntegratorStateMustResolveToSignalObject=off  IntegratorRTWStateStorageClass=Auto  FilterContinuousStateAttributes=''  FilterStateMustResolveToSignalObject=off  FilterRTWStateStorageClass=Auto  DifferentiatorICPrevScaledInput=0  DifferentiatorOutMin=[]  DifferentiatorOutMax=[]  FilterDiffOutCoefMin=[]  FilterDiffOutCoefMax=[]  SumDenOutMin=[]  SumDenOutMax=[]  SumNumOutMin=[]  SumNumOutMax=[]  ReciprocalOutMin=[]  ReciprocalOutMax=[]  DivideOutMin=[]  DivideOutMax=[]  TunerSelectOption=Transfer Function Based (PID Tuner App)
  cfblk8 : simulink/Continuous/PID Controller  Controller=PID  TimeDomain=Discrete-time  SampleTime=-1  IntegratorMethod=Forward Euler  FilterMethod=Forward Euler  Form=Parallel  UseFilter=on  ControllerParametersSource=internal  P=1  I=1  D=0  N=100  InitialConditionSource=internal  InitialConditionForIntegrator=0  InitialConditionForFilter=0  ExternalReset=none  LimitOutput=off  UpperSaturationLimit=inf  LowerSaturationLimit=-inf  LinearizeAsGain=off  AntiWindupMode=none  Kb=1  TrackingMode=off  Kt=1  PParamMin=[]  PParamMax=[]  IParamMin=[]  IParamMax=[]  DParamMin=[]  DParamMax=[]  NParamMin=[]  NParamMax=[]  KbParamMin=[]  KbParamMax=[]  KtParamMin=[]  KtParamMax=[]  POutMin=[]  POutMax=[]  IOutMin=[]  IOutMax=[]  DOutMin=[]  DOutMax=[]  NOutMin=[]  NOutMax=[]  KbOutMin=[]  KbOutMax=[]  KtOutMin=[]  KtOutMax=[]  IntegratorOutMin=[]  IntegratorOutMax=[]  FilterOutMin=[]  FilterOutMax=[]  SumOutMin=[]  SumOutMax=[]  SumI1OutMin=[]  SumI1OutMax=[]  SumI2OutMin=[]  SumI2OutMax=[]  SumI3OutMin=[]  SumI3OutMax=[]  SumDOutMin=[]  SumDOutMax=[]  SaturationOutMin=[]  SaturationOutMax=[]  IntegratorContinuousStateAttributes=''  IntegratorStateMustResolveToSignalObject=off  IntegratorRTWStateStorageClass=Auto  FilterContinuousStateAttributes=''  FilterStateMustResolveToSignalObject=off  FilterRTWStateStorageClass=Auto  DifferentiatorICPrevScaledInput=0  DifferentiatorOutMin=[]  DifferentiatorOutMax=[]  FilterDiffOutCoefMin=[]  FilterDiffOutCoefMax=[]  SumDenOutMin=[]  SumDenOutMax=[]  SumNumOutMin=[]  SumNumOutMax=[]  ReciprocalOutMin=[]  ReciprocalOutMax=[]  DivideOutMin=[]  DivideOutMax=[]  TunerSelectOption=Transfer Function Based (PID Tuner App)
  cfblk9 : DiscreteStateSpace  SampleTime=-1
  cyemi_{1543..1547,1562,1581..1591} (17 alike) : DataTypeConversion  OutDataTypeStr=double
  cfblk2 : Outport
  cfblk13 : Outport  Port=2
  cfblk14 : Outport  Port=3
  wires:
  cfblk8/1 -> cfblk14/1, cyemi_1586/1
  cfblk16/2(cfblk17) -> cfblk13/1, cyemi_1544/1
  cfblk15/2(cfblk17) -> cfblk2/1
  cfblk4/1 -> cyemi_1583/1, cyemi_1589/1
  cfblk12/1 -> cfblk15/Action
  cfblk12/2 -> cfblk16/Action
  cyemi_1543/1 -> cfblk10/1
  cfblk6/1 -> cyemi_1543/1
  cyemi_1544/1 -> cfblk11/1
  cyemi_1545/1 -> cfblk12/1
  cfblk18/1 -> cyemi_1545/1
  cyemi_1546/1 -> cfblk15/1(cfblk1)
  cfblk10/1 -> cyemi_1546/1
  cyemi_1547/1 -> cfblk15/2(cfblk16)
  cfblk19/1 -> cyemi_1547/1
  cyemi_1562/1 -> cfblk16/1(cfblk1)
  cfblk17/1 -> cyemi_1562/1
  cyemi_1581/1 -> cfblk17/1
  cfblk5/1 -> cyemi_1581/1
  cyemi_1582/1 -> cfblk18/1
  cfblk7/1 -> cyemi_1582/1
  cyemi_1583/1 -> cfblk19/1
  cyemi_1584/1 -> cfblk3/1
  cfblk9/1 -> cyemi_1584/1
  cyemi_1585/1 -> cfblk4/1
  cfblk16/1(cfblk2) -> cyemi_1585/1
  cyemi_1586/1 -> cfblk5/1
  cyemi_1587/1 -> cfblk6/1
  cfblk1/1 -> cyemi_1587/1
  cyemi_1588/1 -> cfblk7/1
  cfblk3/1 -> cyemi_1588/1
  cyemi_1589/1 -> cfblk7/2
  cyemi_1590/1 -> cfblk8/1
  cfblk15/1(cfblk2) -> cyemi_1590/1
  cyemi_1591/1 -> cfblk9/1
  cfblk11/1 -> cyemi_1591/1

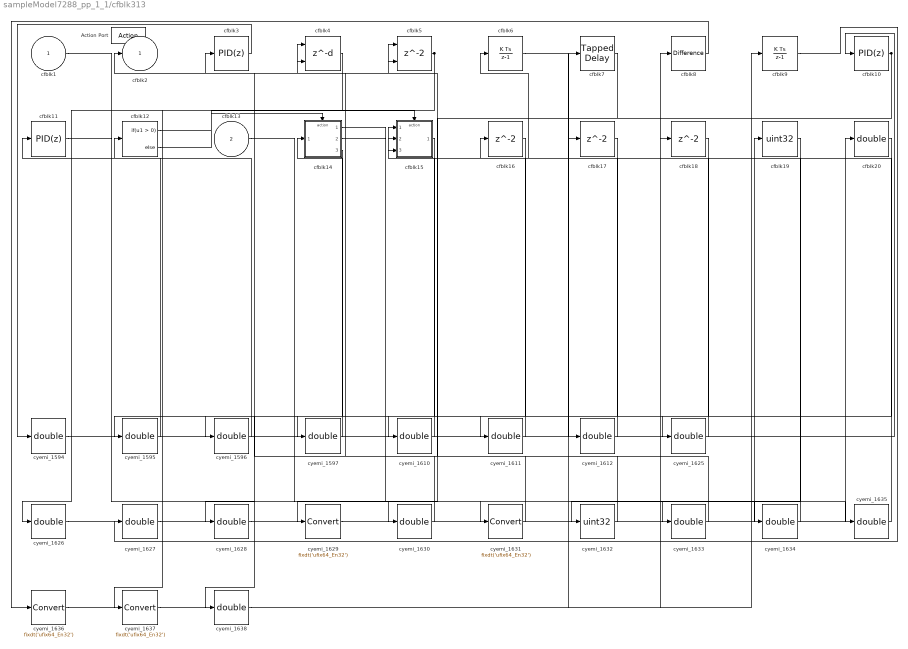
== system sampleModel7288_pp_1_1/cfblk313 ==
  cfblk1 : Inport
  cfblk13 : Inport  Port=2
  Action Port : ActionPort  ActionType=else
  cfblk10 : simulink/Continuous/PID Controller  Controller=PID  TimeDomain=Discrete-time  SampleTime=-1  IntegratorMethod=Forward Euler  FilterMethod=Forward Euler  Form=Parallel  UseFilter=on  ControllerParametersSource=internal  P=1  I=1  D=0  N=100  InitialConditionSource=internal  InitialConditionForIntegrator=0  InitialConditionForFilter=0  ExternalReset=none  LimitOutput=off  UpperSaturationLimit=inf  LowerSaturationLimit=-inf  LinearizeAsGain=off  AntiWindupMode=none  Kb=1  TrackingMode=off  Kt=1  PParamMin=[]  PParamMax=[]  IParamMin=[]  IParamMax=[]  DParamMin=[]  DParamMax=[]  NParamMin=[]  NParamMax=[]  KbParamMin=[]  KbParamMax=[]  KtParamMin=[]  KtParamMax=[]  POutMin=[]  POutMax=[]  IOutMin=[]  IOutMax=[]  DOutMin=[]  DOutMax=[]  NOutMin=[]  NOutMax=[]  KbOutMin=[]  KbOutMax=[]  KtOutMin=[]  KtOutMax=[]  IntegratorOutMin=[]  IntegratorOutMax=[]  FilterOutMin=[]  FilterOutMax=[]  SumOutMin=[]  SumOutMax=[]  SumI1OutMin=[]  SumI1OutMax=[]  SumI2OutMin=[]  SumI2OutMax=[]  SumI3OutMin=[]  SumI3OutMax=[]  SumDOutMin=[]  SumDOutMax=[]  SaturationOutMin=[]  SaturationOutMax=[]  IntegratorContinuousStateAttributes=''  IntegratorStateMustResolveToSignalObject=off  IntegratorRTWStateStorageClass=Auto  FilterContinuousStateAttributes=''  FilterStateMustResolveToSignalObject=off  FilterRTWStateStorageClass=Auto  DifferentiatorICPrevScaledInput=0  DifferentiatorOutMin=[]  DifferentiatorOutMax=[]  FilterDiffOutCoefMin=[]  FilterDiffOutCoefMax=[]  SumDenOutMin=[]  SumDenOutMax=[]  SumNumOutMin=[]  SumNumOutMax=[]  ReciprocalOutMin=[]  ReciprocalOutMax=[]  DivideOutMin=[]  DivideOutMax=[]  TunerSelectOption=Transfer Function Based (PID Tuner App)
  cfblk11 : simulink/Continuous/PID Controller  Controller=PID  TimeDomain=Discrete-time  SampleTime=-1  IntegratorMethod=Forward Euler  FilterMethod=Forward Euler  Form=Parallel  UseFilter=on  ControllerParametersSource=internal  P=1  I=1  D=0  N=100  InitialConditionSource=internal  InitialConditionForIntegrator=0  InitialConditionForFilter=0  ExternalReset=none  LimitOutput=off  UpperSaturationLimit=inf  LowerSaturationLimit=-inf  LinearizeAsGain=off  AntiWindupMode=none  Kb=1  TrackingMode=off  Kt=1  PParamMin=[]  PParamMax=[]  IParamMin=[]  IParamMax=[]  DParamMin=[]  DParamMax=[]  NParamMin=[]  NParamMax=[]  KbParamMin=[]  KbParamMax=[]  KtParamMin=[]  KtParamMax=[]  POutMin=[]  POutMax=[]  IOutMin=[]  IOutMax=[]  DOutMin=[]  DOutMax=[]  NOutMin=[]  NOutMax=[]  KbOutMin=[]  KbOutMax=[]  KtOutMin=[]  KtOutMax=[]  IntegratorOutMin=[]  IntegratorOutMax=[]  FilterOutMin=[]  FilterOutMax=[]  SumOutMin=[]  SumOutMax=[]  SumI1OutMin=[]  SumI1OutMax=[]  SumI2OutMin=[]  SumI2OutMax=[]  SumI3OutMin=[]  SumI3OutMax=[]  SumDOutMin=[]  SumDOutMax=[]  SaturationOutMin=[]  SaturationOutMax=[]  IntegratorContinuousStateAttributes=''  IntegratorStateMustResolveToSignalObject=off  IntegratorRTWStateStorageClass=Auto  FilterContinuousStateAttributes=''  FilterStateMustResolveToSignalObject=off  FilterRTWStateStorageClass=Auto  DifferentiatorICPrevScaledInput=0  DifferentiatorOutMin=[]  DifferentiatorOutMax=[]  FilterDiffOutCoefMin=[]  FilterDiffOutCoefMax=[]  SumDenOutMin=[]  SumDenOutMax=[]  SumNumOutMin=[]  SumNumOutMax=[]  ReciprocalOutMin=[]  ReciprocalOutMax=[]  DivideOutMin=[]  DivideOutMax=[]  TunerSelectOption=Transfer Function Based (PID Tuner App)
  cfblk12 : If  SampleTime=1
  cfblk14 : Subsystem  TreatAsAtomicUnit=on
  cfblk15 : Subsystem  TreatAsAtomicUnit=on
  cfblk16 : Delay
  cfblk17 : Delay
  cfblk18 : Delay
  cfblk19 : DataTypeConversion  OutDataTypeStr=uint32
  cfblk20 : DataTypeConversion  OutDataTypeStr=double
  cfblk3 : simulink/Continuous/PID Controller  Controller=PID  TimeDomain=Discrete-time  SampleTime=-1  IntegratorMethod=Forward Euler  FilterMethod=Forward Euler  Form=Parallel  UseFilter=on  ControllerParametersSource=internal  P=1  I=1  D=0  N=100  InitialConditionSource=internal  InitialConditionForIntegrator=0  InitialConditionForFilter=0  ExternalReset=none  LimitOutput=off  UpperSaturationLimit=inf  LowerSaturationLimit=-inf  LinearizeAsGain=off  AntiWindupMode=none  Kb=1  TrackingMode=off  Kt=1  PParamMin=[]  PParamMax=[]  IParamMin=[]  IParamMax=[]  DParamMin=[]  DParamMax=[]  NParamMin=[]  NParamMax=[]  KbParamMin=[]  KbParamMax=[]  KtParamMin=[]  KtParamMax=[]  POutMin=[]  POutMax=[]  IOutMin=[]  IOutMax=[]  DOutMin=[]  DOutMax=[]  NOutMin=[]  NOutMax=[]  KbOutMin=[]  KbOutMax=[]  KtOutMin=[]  KtOutMax=[]  IntegratorOutMin=[]  IntegratorOutMax=[]  FilterOutMin=[]  FilterOutMax=[]  SumOutMin=[]  SumOutMax=[]  SumI1OutMin=[]  SumI1OutMax=[]  SumI2OutMin=[]  SumI2OutMax=[]  SumI3OutMin=[]  SumI3OutMax=[]  SumDOutMin=[]  SumDOutMax=[]  SaturationOutMin=[]  SaturationOutMax=[]  IntegratorContinuousStateAttributes=''  IntegratorStateMustResolveToSignalObject=off  IntegratorRTWStateStorageClass=Auto  FilterContinuousStateAttributes=''  FilterStateMustResolveToSignalObject=off  FilterRTWStateStorageClass=Auto  DifferentiatorICPrevScaledInput=0  DifferentiatorOutMin=[]  DifferentiatorOutMax=[]  FilterDiffOutCoefMin=[]  FilterDiffOutCoefMax=[]  SumDenOutMin=[]  SumDenOutMax=[]  SumNumOutMin=[]  SumNumOutMax=[]  ReciprocalOutMin=[]  ReciprocalOutMax=[]  DivideOutMin=[]  DivideOutMax=[]  TunerSelectOption=Transfer Function Based (PID Tuner App)
  cfblk4 : Delay  DelayLengthSource=Input port
      settings: InputPortMap=u0,p1
  cfblk5 : Delay  ShowEnablePort=on
      settings: InputPortMap=u0,e6
  cfblk6 : DiscreteIntegrator  SampleTime=-1  OutDataTypeStr=double  ICPrevOutput=DiscIntNeverNeededParam  ICPrevScaledInput=DiscIntNeverNeededParam
  cfblk7 : simulink/Discrete/Tapped Delay  vinit=0.0  samptime=-1  NumDelays=1  DelayOrder=Oldest  includeCurrent=off
  cfblk8 : simulink/Discrete/Difference  ICPrevInput=0.0  OutMin=[]  OutMax=[]  OutDataTypeStr=fixdt('ufix64_En32')  OutputDataTypeScalingMode=Specify via dialog  OutDataType=fixdt('ufix64_En32')  OutScaling=[]  DoSatur=off
  cfblk9 : DiscreteIntegrator  SampleTime=-1  OutDataTypeStr=double  ICPrevOutput=DiscIntNeverNeededParam  ICPrevScaledInput=DiscIntNeverNeededParam
  cyemi_{1594..1597,1610..1612,1625..1628,1630,1633..1635,1638} (16 alike) : DataTypeConversion  OutDataTypeStr=double
  cyemi_{1629,1631,1636..1637} (4 alike) : DataTypeConversion  OutDataTypeStr=fixdt('ufix64_En32')
  cyemi_1632 : DataTypeConversion  OutDataTypeStr=uint32
  cfblk2 : Outport
  wires:
  cfblk5/1 -> cfblk2/1, cyemi_1626/1
  cfblk10/1 -> cyemi_1596/1, cyemi_1597/1
  cfblk12/1 -> cfblk14/Action
  cfblk12/2 -> cfblk15/Action
  cyemi_1594/1 -> cfblk10/1
  cfblk3/1 -> cyemi_1594/1
  cyemi_1595/1 -> cfblk11/1
  cfblk14/3(cfblk10) -> cyemi_1595/1
  cyemi_1596/1 -> cfblk12/1
  cyemi_1597/1 -> cfblk14/1(cfblk1)
  cyemi_1610/1 -> cfblk15/1(cfblk1)
  cfblk17/1 -> cyemi_1610/1
  cyemi_1611/1 -> cfblk15/2(cfblk14)
  cfblk18/1 -> cyemi_1611/1
  cyemi_1612/1 -> cfblk15/3(cfblk15)
  cfblk6/1 -> cyemi_1612/1
  cyemi_1625/1 -> cfblk16/1
  cfblk20/1 -> cyemi_1625/1
  cyemi_1626/1 -> cfblk17/1
  cyemi_1627/1 -> cfblk18/1
  cfblk9/1 -> cyemi_1627/1
  cyemi_1628/1 -> cfblk19/1
  cfblk16/1 -> cyemi_1628/1
  cyemi_1629/1 -> cfblk20/1
  cfblk7/1 -> cyemi_1629/1
  cyemi_1630/1 -> cfblk3/1
  cfblk1/1 -> cyemi_1630/1
  cyemi_1631/1 -> cfblk4/1
  cfblk14/1(cfblk2) -> cyemi_1631/1
  cyemi_1632/1 -> cfblk4/2
  cfblk19/1 -> cyemi_1632/1
  cyemi_1633/1 -> cfblk5/1
  cfblk11/1 -> cyemi_1633/1
  cyemi_1634/1 -> cfblk5/2
  cfblk14/2(cfblk9) -> cyemi_1634/1
  cyemi_1635/1 -> cfblk6/1
  cfblk13/1 -> cyemi_1635/1
  cyemi_1636/1 -> cfblk7/1
  cfblk8/1 -> cyemi_1636/1
  cyemi_1637/1 -> cfblk8/1
  cfblk4/1 -> cyemi_1637/1
  cyemi_1638/1 -> cfblk9/1
  cfblk15/1(cfblk2) -> cyemi_1638/1

== system sampleModel7288_pp_1_1/cfblk314 ==
  cfblk1 : Inport
  cfblk7 : Inport  Port=2
  cfblk8 : Inport  Port=3
  Action Port : ActionPort  ActionType=then
  cfblk10 : Subsystem  TreatAsAtomicUnit=on
  cfblk11 : Subsystem  TreatAsAtomicUnit=on
  cfblk12 : Delay
  cfblk13 : Delay
  cfblk3 : DiscreteTransferFcn
  cfblk4 : simulink/Discrete/Transfer Fcn Real Zero  ZeroZ=0.75  ICPrevInput=0.0  DoSatur=off
      settings: SourceProductName=Simulink  SourceProductBaseCode=SL
  cfblk5 : simulink/Discrete/Difference  ICPrevInput=0.0  OutMin=[]  OutMax=[]  OutDataTypeStr=double  OutputDataTypeScalingMode=double  OutDataType=fixdt(1, 16)  OutScaling=2^-10  DoSatur=off
  cfblk6 : If  SampleTime=1
  cyemi_{1642..1644,1654,1663..1668} (10 alike) : DataTypeConversion  OutDataTypeStr=double
  cfblk2 : Outport
  cfblk9 : Outport  Port=2
  wires:
  cfblk1/1 -> cfblk9/1, cyemi_1644/1
  cfblk11/2(cfblk9) -> cfblk2/1
  cfblk6/1 -> cfblk10/Action
  cfblk6/2 -> cfblk11/Action
  cyemi_1642/1 -> cfblk10/1(cfblk1)
  cfblk3/1 -> cyemi_1642/1
  cyemi_1643/1 -> cfblk10/2(cfblk10)
  cfblk12/1 -> cyemi_1643/1
  cyemi_1644/1 -> cfblk10/3(cfblk11)
  cyemi_1654/1 -> cfblk11/1(cfblk1)
  cfblk8/1 -> cyemi_1654/1
  cyemi_1663/1 -> cfblk12/1
  cfblk5/1 -> cyemi_1663/1
  cyemi_1664/1 -> cfblk13/1
  cfblk11/1(cfblk2) -> cyemi_1664/1
  cyemi_1665/1 -> cfblk3/1
  cfblk7/1 -> cyemi_1665/1
  cyemi_1666/1 -> cfblk4/1
  cfblk10/1(cfblk2) -> cyemi_1666/1
  cyemi_1667/1 -> cfblk5/1
  cfblk4/1 -> cyemi_1667/1
  cyemi_1668/1 -> cfblk6/1
  cfblk13/1 -> cyemi_1668/1

== system sampleModel7288_pp_1_1/cfblk315 ==
  cfblk1 : Inport
  Action Port : ActionPort  ActionType=else
  cfblk10 : Subsystem  TreatAsAtomicUnit=on
  cfblk11 : Delay
  cfblk3 : simulink/Discrete/Tapped Delay  vinit=0.0  samptime=-1  NumDelays=1  DelayOrder=Oldest  includeCurrent=off
  cfblk4 : simulink/Discrete/Tapped Delay  vinit=0.0  samptime=-1  NumDelays=1  DelayOrder=Oldest  includeCurrent=off
  cfblk5 : DiscreteStateSpace  SampleTime=-1
  cfblk6 : simulink/Discrete/Transfer Fcn Lead or Lag  PoleZ=0.95  ZeroZ=0.75  ICPrevOutput=0.0  ICPrevInput=0.0  DoSatur=off
      settings: SourceProductName=Simulink  SourceProductBaseCode=SL
  cfblk7 : If  SampleTime=1
  cfblk9 : Subsystem  TreatAsAtomicUnit=on
  cyemi_{1670..1672,1685..1691} (10 alike) : DataTypeConversion  OutDataTypeStr=double
  cfblk2 : Outport
  cfblk8 : Outport  Port=2
  wires:
  cfblk1/1 -> cyemi_1689/1, cyemi_1690/1
  cfblk10/1(cfblk2) -> cfblk8/1
  cfblk5/1 -> cfblk2/1, cyemi_1685/1
  cfblk7/1 -> cfblk9/Action
  cfblk7/2 -> cfblk10/Action
  cyemi_1670/1 -> cfblk10/1(cfblk1)
  cfblk9/1(cfblk2) -> cyemi_1670/1
  cyemi_1671/1 -> cfblk10/2(cfblk12)
  cfblk9/2(cfblk7) -> cyemi_1671/1
  cyemi_1672/1 -> cfblk10/3(cfblk13)
  cfblk11/1 -> cyemi_1672/1
  cyemi_1685/1 -> cfblk11/1
  cyemi_1686/1 -> cfblk3/1
  cfblk10/2(cfblk14) -> cyemi_1686/1
  cyemi_1687/1 -> cfblk4/1
  cfblk3/1 -> cyemi_1687/1
  cyemi_1688/1 -> cfblk5/1
  cfblk4/1 -> cyemi_1688/1
  cyemi_1689/1 -> cfblk6/1
  cyemi_1690/1 -> cfblk7/1
  cyemi_1691/1 -> cfblk9/1(cfblk1)
  cfblk6/1 -> cyemi_1691/1
